simulink model "MCCE"  (R2022b)
settings: Solver=VariableStepAuto  StartTime=0.0  StopTime=240  RelTol=1e-3
values from neighbouring files (symbols this model uses):
  A_obsv = [0 0 0 0 0 0 0 0 0 0 0 0 ... (144 elements, 12x12)]    [L1_result.mat]    (also in L2_results.mat; Run_file.m = kron(eye(num_agents),A(0.1,pi/6)); result.mat)
  adj = [0 0 0 1 0 0 0 0 0 0 0 0 ... (144 elements, 12x12)]    [L1_result.mat]    (also in L2_results.mat; Run_file.m = kron(diag(diag(L))-L, eye(n_states)); Static_test.m = kron(diag(diag(L))-L, eye(n_states)); distributed_L1_minimization.m = kron(in_degree-L, eye(n_states)))
  C = [1  0  0; 0  1  0]    [L1_result.mat]    (also in L2_results.mat; Run_file.m = eye(2,n_states); Test_static_estimation.m = [C1; C2; C3]; result.mat)
  C_block = [1 0 0 0 0 0 0 0 0 1 0 0 ... (96 elements, 8x12)]    [L1_result.mat]    (also in L2_results.mat; Run_file.m = blkdiag(C,C,C,C); result.mat)
  goalLoc = [12 3]    [L1_result.mat]    (also in L2_results.mat; Run_file.m; result.mat)
  in_degree = [1 2 1 2]    [L1_result.mat]    (also in L2_results.mat; Run_file.m = diag(L); Static_test.m = diag(L); distributed_L1_minimization.m = diag(diag(L)))
  L_bar = [1 0 0 -1 0 0 0 0 0 0 0 0 ... (144 elements, 12x12)]    [L1_result.mat]    (also in L2_results.mat; Run_file.m = kron(L, eye(n_states)); Static_test.m = kron(L, eye(n_states)); distributed_L1_minimization.m = kron(L, eye(n_states)))
  L_obsv_blk = [2.55458080484 -0.951826184038 -20.5459723977 0 0 0 0 0 0 0 0 0 ... (96 elements, 12x8)]    [L1_result.mat]    (also in L2_results.mat; Run_file.m = kron(eye(num_agents),L_obsv); result.mat)
  max_iter = 500    [L1_result.mat]    (also in L2_results.mat; Run_file.m; Static_test.m; Test_static_estimation.m = 1000)
  n_meas = 3    [L1_result.mat]    (also in L2_results.mat; Run_file.m; Static_test.m; Test_static_estimation.m = size(C,1))
  n_states = 3    [L1_result.mat]    (also in L2_results.mat; Run_file.m; Static_test.m; Test_static_estimation.m = 4)
  num_agents = 4    [L1_result.mat]    (also in L2_results.mat; Run_file.m; Static_test.m; Test_static_estimation.m = 3)
  plane = 2.282825    [L1_result.mat]    (also in L2_results.mat; Run_file.m; Static_test.m; result.mat)
  R1 = [0.996940014454  -0.0778516423796  -0.00705190468025; -0.0666274822561  -0.799083626549  -0.597516641098; 0.0408825902926  0.596158099466  -0.801825501123]    [L1_result.mat]    (also in L2_results.mat; Run_file.m = extrinsics{1}.R)
  R_cent = [0.996940014454 -0.0666274822561 0.0408825902926 0.927521105169 0.250159120838 -0.277713906256 -0.758684572339 0.40310063072 -0.511769089735 -0.9827802276 -0.137977656748 0.122903175207 ... (36 elements, 12x3)]    [L1_result.mat]    (also in L2_results.mat; Run_file.m = zeros(num_agents*n_meas,n_states); Static_test.m = zeros(num_agents*n_meas,n_states); result.mat)
  R_dist =     [L1_result.mat]    (also in L2_results.mat; Run_file.m = cell(1,num_agents); Static_test.m = cell(1,num_agents); result.mat)
  simpleMap = [1 1 1 1 1 1 1 1 1 1 1 1 ... (702 elements, 26x27)]    [L1_result.mat]    (also in L2_results.mat; result.mat)
  startLoc = [5 5]    [L1_result.mat]    (also in L2_results.mat; Run_file.m; result.mat)
  t_cent = [0.189277412265 -0.439756767494 3.20420262901 -0.721662687527 -0.239717224399 4.46829798951 -1.30366493998 -1.32418253125 5.13323005858 0.209514587747 -0.738276322765 4.88530151004]    [L1_result.mat]    (also in L2_results.mat; Run_file.m = zeros(num_agents*n_meas,1); result.mat)
  z0 = [1 0 0 1 2 0 1 4 0 1 6 0]    [L1_result.mat]    (also in L2_results.mat; Run_file.m = [1;0;0; result.mat)
libraries: robotmobilelib x1, robotalgslib x1
settings Model: Creator=Abelb  LastModifiedBy=Abelb

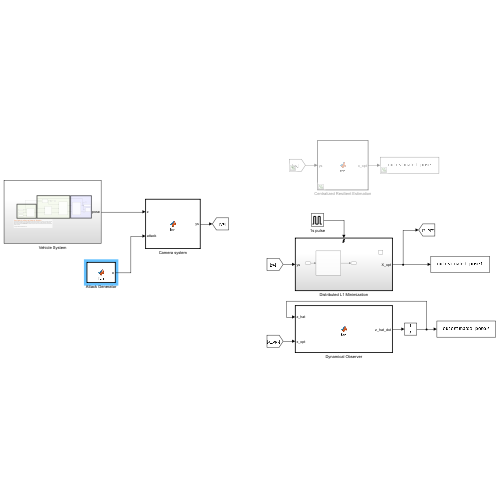
[thumbnail: Simulink's stored preview of the top-level diagram]
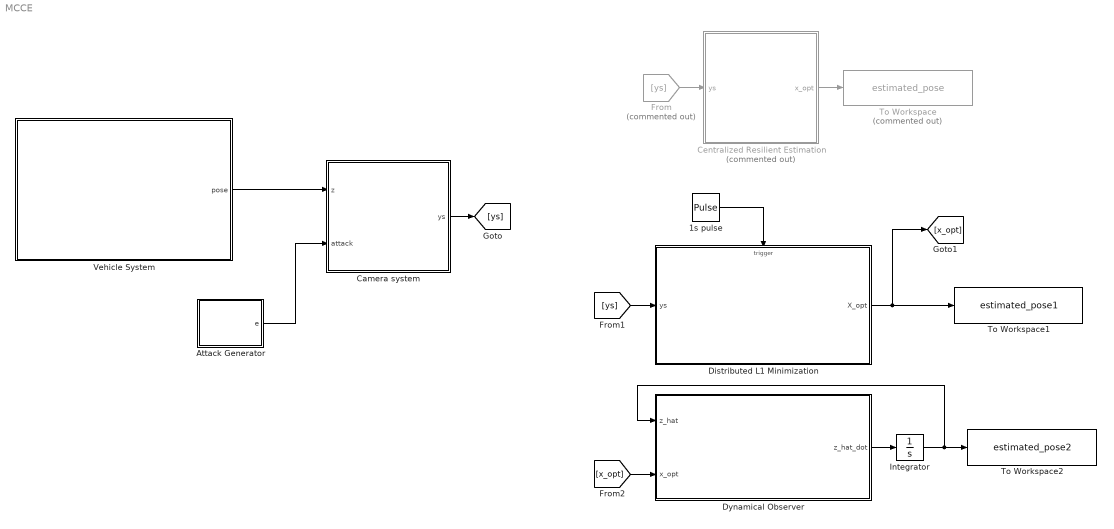
== system MCCE ==
  1s pulse : DiscretePulseGenerator  PulseType=Time based  Period=1  PulseWidth=5
  Attack Generator : MATLAB Function  TreatAsAtomicUnit=on
  Camera system : MATLAB Function  TreatAsAtomicUnit=on
  Centralized Resilient Estimation : MATLAB Function  Commented=on  TreatAsAtomicUnit=on
  Distributed L1 Minimization : Subsystem
  Dynamical Observer : MATLAB Function  TreatAsAtomicUnit=on
  From : From  Commented=on  GotoTag=ys
  Integrator : Integrator  InitialCondition=z0
  To Workspace : ToWorkspace  Commented=on  VariableName=estimated_pose  SampleTime=-1
  To Workspace1 : ToWorkspace  VariableName=estimated_pose1  SampleTime=-1
  To Workspace2 : ToWorkspace  VariableName=estimated_pose2  SampleTime=-1
  Vehicle System : Subsystem
  wires:
  Vehicle System/1(pose) -> Camera system/1(z)
  Attack Generator/1(e) -> Camera system/2(attack)
  Centralized Resilient Estimation/1(x_opt) -> To Workspace/1
  Camera system/1(ys) -> [ys]
  From/1 -> Centralized Resilient Estimation/1(ys)
  1s pulse/1 -> Distributed L1 Minimization/Trigger
  [ys] -> Distributed L1 Minimization/1(ys)
  Distributed L1 Minimization/1(X_opt) -> [x_opt], To Workspace1/1
  [x_opt] -> Dynamical Observer/2(x_opt)
  Dynamical Observer/1(z_hat_dot) -> Integrator/1
  Integrator/1 -> To Workspace2/1, Dynamical Observer/1(z_hat)

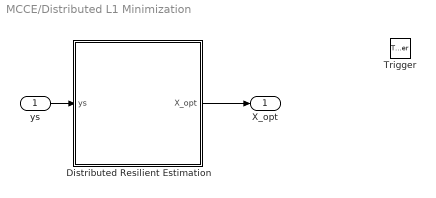
== system MCCE/Distributed L1 Minimization ==
  ys : Inport
  Trigger : TriggerPort  VariantControl=(inherit)  PortDimensions=1
  Distributed Resilient Estimation : MATLAB Function  TreatAsAtomicUnit=on
  X_opt : Outport
  wires:
  ys/1 -> Distributed Resilient Estimation/1(ys)
  Distributed Resilient Estimation/1(X_opt) -> X_opt/1

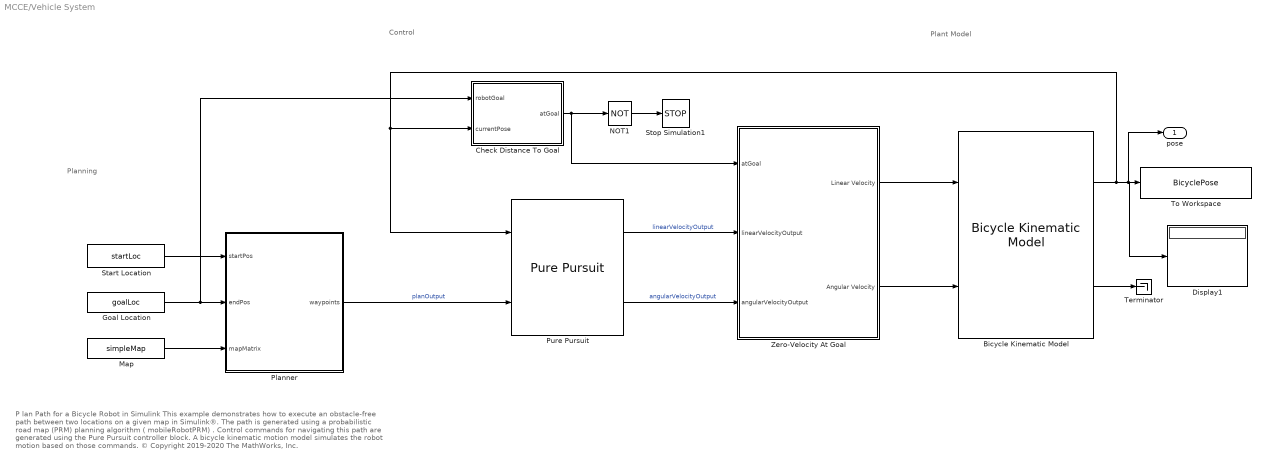
== system MCCE/Vehicle System ==
  note: Planning
  note: P lan Path for a Bicycle Robot in Simulink
      | This example demonstrates how to execute an obstacle-free path between two locations on a given map in Simulink®. The path is generated using a probabilistic road map (PRM) planning algorithm ( mobileRobotPRM) . Control commands for navigating this path are generated using the Pure Pursuit controller block. A bicycle kinematic motion model simulates the robot motion based on those commands.
      |
      | © Copyright 2019-2020 The MathWorks, Inc.
  note: Plant Model
  note: Control
  Bicycle Kinematic Model : robotmobilelib/Bicycle Kinematic Model  VehicleInputs=Vehicle Speed & Heading Angular Velocity  WheelBase=WheelBase  VehicleSpeedRange=constraint_velocity  MaxSteeringAngle=constraint_steering  InitialState=[5; 5; 0]  SimulateUsing=Interpreted execution
  Check Distance To Goal : Subsystem
  Display1 : Display
  Goal Location : Constant  Value=goalLoc
  Map : Constant  Value=simpleMap
  NOT1 : Logic  Operator=NOT  IconShape=distinctive  AllPortsSameDT=off  OutDataTypeStr=boolean
  Planner : MATLAB Function  TreatAsAtomicUnit=on
  Pure Pursuit : robotalgslib/Pure Pursuit  DesiredLinearVelocity=vd  MaxAngularVelocity=constraint_steering  LookaheadDistance=0.5  TargetDirPort=off  SimulateUsing=Code generation
  Start Location : Constant  Value=startLoc
  Stop Simulation1 : Stop
  Terminator : Terminator
  To Workspace : ToWorkspace  VariableName=BicyclePose  SampleTime=-1
  Zero-Velocity At Goal : Subsystem
  pose : Outport
  wires:
  Bicycle Kinematic Model/2 -> Terminator/1
  Zero-Velocity At Goal/1(Linear Velocity) -> Bicycle Kinematic Model/1
  Pure Pursuit/1 -> Zero-Velocity At Goal/2(linearVelocityOutput)  "linearVelocityOutput"
  Map/1 -> Planner/3(mapMatrix)
  Start Location/1 -> Planner/1(startPos)
  Bicycle Kinematic Model/1 -> Pure Pursuit/1, Check Distance To Goal/2(currentPose), pose/1, Display1/1, To Workspace/1
  Zero-Velocity At Goal/2(Angular Velocity) -> Bicycle Kinematic Model/2
  NOT1/1 -> Stop Simulation1/1
  Check Distance To Goal/1(atGoal) -> Zero-Velocity At Goal/1(atGoal), NOT1/1
  Planner/1(waypoints) -> Pure Pursuit/2  "planOutput"
  Goal Location/1 -> Check Distance To Goal/1(robotGoal), Planner/2(endPos)
  Pure Pursuit/2 -> Zero-Velocity At Goal/3(angularVelocityOutput)  "angularVelocityOutput"

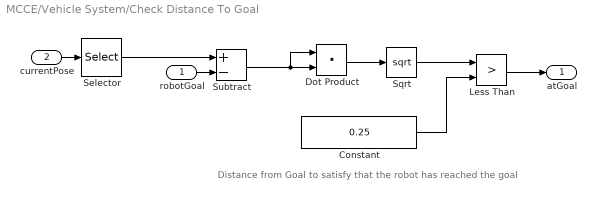
== system MCCE/Vehicle System/Check Distance To Goal ==
  note: Distance from Goal to satisfy that the robot has reached the goal
  robotGoal : Inport
  currentPose : Inport  Port=2
  Constant : Constant  Value=0.25
  Dot Product : DotProduct  OutDataTypeStr=Inherit: Inherit via internal rule
  Less Than : RelationalOperator  Operator=>  OutDataTypeStr=boolean  RndMeth=Simplest  InputSameDT=off
  Selector : Selector  InputPortWidth=3  IndexOptions=Index vector (dialog)  Indices=[1 2]  OutputSizes=1
  Sqrt : Sqrt
  Subtract : Sum  Inputs=+-
  atGoal : Outport
  wires:
  robotGoal/1 -> Subtract/2
  Dot Product/1 -> Sqrt/1
  Constant/1 -> Less Than/2
  currentPose/1 -> Selector/1
  Less Than/1 -> atGoal/1
  Sqrt/1 -> Less Than/1
  Subtract/1 -> Dot Product/1, Dot Product/2
  Selector/1 -> Subtract/1

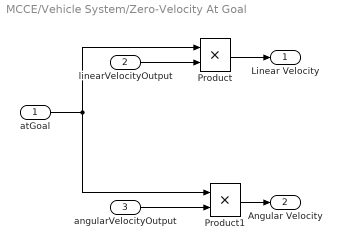
== system MCCE/Vehicle System/Zero-Velocity At Goal ==
  atGoal : Inport
  linearVelocityOutput : Inport  Port=2
  angularVelocityOutput : Inport  Port=3
  Product : Product
  Product1 : Product
  Linear Velocity : Outport  OutDataTypeStr=double
  Angular Velocity : Outport  Port=2  OutDataTypeStr=double
  wires:
  atGoal/1 -> Product1/1, Product/1
  angularVelocityOutput/1 -> Product1/2
  linearVelocityOutput/1 -> Product/2
  Product/1 -> Linear Velocity/1
  Product1/1 -> Angular Velocity/1

== matlab function MCCE/Vehicle System/Planner ==
  settings: updateMethod=DISCRETE
  data: startPos input size=[1 2]; endPos input size=[1 2]; waypoints output size=[100 2]; mapMatrix input
function waypoints = planning(startPos, endPos, mapMatrix)

persistent waypointsInternal
persistent prevStartPos
persistent prevEndPos

% Set constant parameters
maxNumNodes = 100;

% Initialize persistent variables that are used downstream
if isempty(prevStartPos)
    prevStartPos = startPos;
end

if isempty(prevEndPos)
    prevEndPos = endPos;
end

isNewPath = (~isequal(prevStartPos, startPos) || ~isequal(prevEndPos, endPos));

if isempty(waypointsInternal) || isNewPath
    % Two conditions in which waypoints must be set: they are not yet
    % initialized, or they are initialized, but the current start and end
    % do not match those used to generate the previous set of waypoints
    [waypointsInternal] = planPath(mapMatrix, maxNumNodes, startPos, endPos);
end

% Update the outputs
waypoints = waypointsInternal;

% Update the persistent variables that indicate previous state
prevStartPos = startPos;
prevEndPos = endPos;

%% Helper Function

function wayPoints = planPath(mapMatrix, maxNodes, startPos, endPos)
    
    % Create a probabilistic roadmap
    map = binaryOccupancyMap(mapMatrix);
    prm = mobileRobotPRM(map, maxNodes);
    
    % Find a path between two points
    xy = findpath(prm, startPos, endPos);
    wayPoints = repmat(endPos, maxNodes, 1);
    
    % Number of nodes that are actually used
    numNodes = length(xy);
    wayPoints(1:numNodes,:) = xy;    

end

end

== matlab function MCCE/Camera system ==
  data: z input; ys output; attack input; n_meas parameter; num_agents parameter; R_cent parameter; plane parameter; t_cent parameter; C parameter
function ys = fcn(z,attack, n_meas, num_agents, R_cent, plane, t_cent,C)

%% vehicle measurement
x = C*z;

%% camera sensing
ys = zeros(num_agents*n_meas,1);
% for cam=1:num_agents
%     R = extrinsics{cam}.R;
%     t = extrinsics{cam}.Translation';
%     ys((cam-1)*n_meas+1:cam*n_meas) = R * x_w + t;
% end
ys(:) = R_cent*[x; plane]+t_cent;


%% attack injection
ys = ys+attack;

== matlab function MCCE/Centralized Resilient Estimation ==
  data: ys input; x_opt output; R_cent parameter; t_cent parameter; n_states parameter; n_meas parameter; num_agents parameter
function x_opt = fcn(ys, R_cent, t_cent, n_states, n_meas,num_agents)

%% L1 minimization
coder.extrinsic('L1_minimization');
x_opt = zeros(n_states,1);
x_opt(:) = L1_minimization(R_cent, ys-t_cent, n_meas*num_agents, n_states);

%% dynamical estimation

== matlab function MCCE/Distributed L1 Minimization/Distributed Resilient Estimation ==
  data: ys input; X_opt output; R_dist parameter; t_cent parameter; n_states parameter; n_meas parameter; num_agents parameter; in_degree parameter; max_iter parameter; L_bar parameter; adj parameter
function X_opt = fcn(ys, R_dist, t_cent, n_states, n_meas,num_agents, in_degree, max_iter, L_bar, adj)

%% distributed L1 minimization
coder.extrinsic('L1_minimization');
coder.extrinsic('distributed_L1_minimization');

ys = ys - t_cent;
% y  = cell(1,num_agents);
% for i_agent = 1:num_agents
%     y{1,i_agent} = ys(n_meas*(i_agent-1)+1:n_meas*i_agent);
% end

%% Local L1 optimization
x1 = L1_minimization(R_dist{1}, ys(1:n_meas), n_meas, n_states);
x2 = L1_minimization(R_dist{2}, ys(n_meas+1:2*n_meas), n_meas, n_states);
x3 = L1_minimization(R_dist{3}, ys(2*n_meas+1:3*n_meas), n_meas, n_states);
x4 = L1_minimization(R_dist{4}, ys(3*n_meas+1:4*n_meas), n_meas, n_states);
x0 = [x1; x2; x3;x4];


%%
y = {ys(1:n_meas), ys(n_meas+1:n_meas*2), ys(n_meas*2+1:n_meas*3), ys(n_meas*3+1:n_meas*4)};

X_opt = zeros(num_agents*n_states,1);
X_opt(:) = distributed_L1_minimization(R_dist, y, in_degree, L_bar, adj, n_states, num_agents, max_iter,x0);
%% dynamical estimation

== matlab function MCCE/Dynamical Observer ==
  data: z_hat input; x_opt input; z_hat_dot output; C_block parameter; L_obsv_blk parameter; A_obsv parameter
function z_hat_dot = fcn(z_hat, x_opt, C_block, L_obsv_blk, A_obsv)

x = [x_opt(1:2); x_opt(4:5); x_opt(7:8); x_opt(10:11)];
z_hat_dot = A_obsv*z_hat + L_obsv_blk*(x - C_block*z_hat);

== matlab function MCCE/Attack Generator ==
  data: e output; n_meas parameter; num_agents parameter; R1 parameter; n_states parameter
function e = fcn(n_meas, num_agents, R1, n_states)

% num_attack = 2;
% sparse_loc = [1,2];
% e = zeros(n_meas*num_agents,1);
% e(sparse_loc) = 2*rand(num_attack,1);

e1 = R1*2*rand(n_states,1);
e = zeros(n_meas*num_agents,1);
e(1:3) = e1;
